simulink model "drone"  (Simulink 6.1)
settings: Solver=ode5  StartTime=0.0  StopTime=90  FixedStep=1e-3  RelTol=1e-3
values from neighbouring files (symbols this model uses):
  Aerodynamique =     [Test en vol.mat]
  Correcteur =     [Test en vol.mat]
  Mecanique =     [Test en vol.mat]
libraries: mblibv1 x43, simulink x26, aerolibtransform2 x4, electricdrivelib x1
(part 1 of 2)
settings Model: LastModifiedBy=Vincent
settings OptimizationCC: InlineParams=on
settings DebuggingCC: SolverPrmCheckMsg=warning
settings SimMechanicsCC: VisOnUpdateDiagram=on  VisDuringSimulation=on

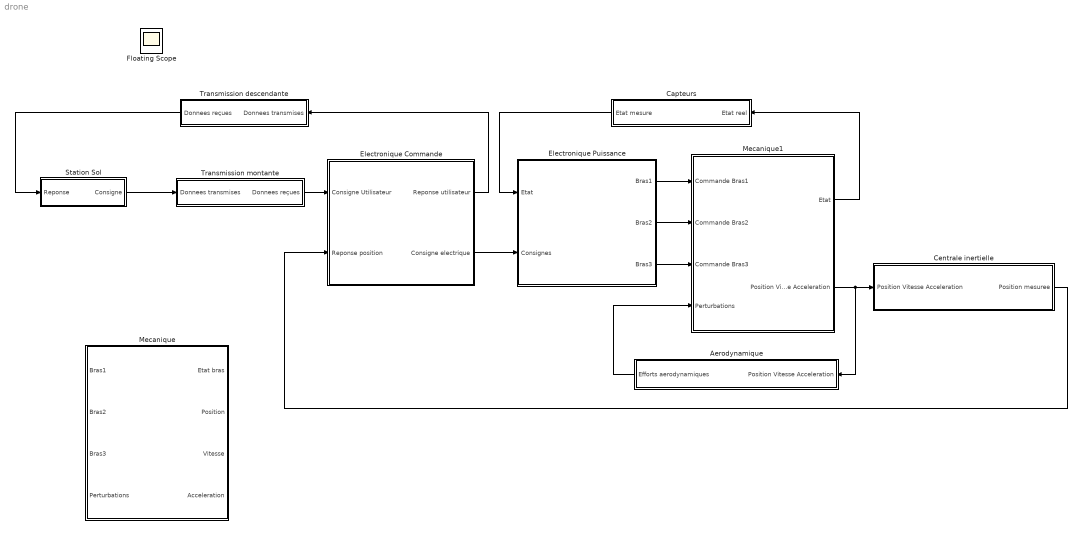
== system drone ==
  Aerodynamique : Subsystem  Orientation=left
  Capteurs : Subsystem  Orientation=left
  Centrale inertielle : Subsystem
  Electronique Commande : Subsystem
  Electronique Puissance : Subsystem
  Mecanique : Subsystem
  Mecanique1 : Subsystem
  Station Sol : Subsystem
  Transmission descendante : Subsystem  Orientation=left
  Transmission montante : Subsystem
  Floating Scope : Scope
      settings: Floating=on
  wires:
  Station Sol/1(Consigne) -> Transmission montante/1(Donnees transmises)
  Centrale inertielle/1(Position mesuree) -> Electronique Commande/2(Reponse position)
  Electronique Puissance/1(Bras1) -> Mecanique1/1(Commande Bras1)
  Electronique Puissance/3(Bras3) -> Mecanique1/3(Commande Bras3)
  Electronique Puissance/2(Bras2) -> Mecanique1/2(Commande Bras2)
  Electronique Commande/2(Consigne electrique) -> Electronique Puissance/2(Consignes)
  Aerodynamique/1(Efforts aerodynamiques) -> Mecanique1/4(Perturbations)
  Mecanique1/1(Etat) -> Capteurs/1(Etat reel)
  Capteurs/1(Etat mesure) -> Electronique Puissance/1(Etat)
  Transmission montante/1(Donnees reçues) -> Electronique Commande/1(Consigne Utilisateur)
  Electronique Commande/1(Reponse utilisateur) -> Transmission descendante/1(Donnees transmises)
  Transmission descendante/1(Donnees reçues) -> Station Sol/1(Reponse)
  Mecanique1/2(Position Vitesse Acceleration) -> Centrale inertielle/1(Position Vitesse Acceleration), Aerodynamique/1(Position Vitesse Acceleration)

== system drone/Aerodynamique ==
  Position Vitesse Acceleration : Inport  Port=1  LatchInput=off
  Bus Creator : BusCreator  DialogController=Simulink.DDGSource_Bus  Inputs=2
  Bus Selector : BusSelector  DialogController=Simulink.DDGSource_Bus  OutputSignals=x'y'z',pqr
  Coef frottement : Gain  Gain=-1*Aerodynamique.Resistance.F
  "Coef frottement " : Gain  Gain=-1*Aerodynamique.Resistance.C
  Efforts aerodynamiques : Outport
      settings: BusObject=perturbations
  wires:
  Position Vitesse Acceleration/1 -> Bus Selector/1
  Bus Selector/1 -> Coef frottement/1  "<x'y'z'>"
  Bus Selector/2 -> "Coef frottement "/1  "<pqr>"
  Coef frottement/1 -> Bus Creator/1  "forces aero"
  "Coef frottement "/1 -> Bus Creator/2  "couples aero"
  Bus Creator/1 -> Efforts aerodynamiques/1

== system drone/Capteurs ==
  Etat reel : Inport  Port=1  LatchInput=off
  Etat mesure : Outport
      settings: BusObject=perturbations
  wires:
  Etat reel/1 -> Etat mesure/1

== system drone/Centrale inertielle ==
  Position Vitesse Acceleration : Inport  Port=1  LatchInput=off
      settings: BusObject=couples_moteurs
  Bus Creator : BusCreator  DialogController=Simulink.DDGSource_Bus  Inputs=2
  Bus Selector : BusSelector  DialogController=Simulink.DDGSource_Bus  OutputSignals=xyz,dcm
  Direction Cosine Matrix  to Quaternions1 : aerolibtransform2/Direction Cosine Matrix  to Quaternions
  Position mesuree : Outport
      settings: BusObject=reponse_generale
  wires:
  Position Vitesse Acceleration/1 -> Bus Selector/1
  Bus Selector/2 -> Direction Cosine Matrix  to Quaternions1/1  "<dcm>"
  Bus Selector/1 -> Bus Creator/1  "<xyz>"
  Direction Cosine Matrix  to Quaternions1/1 -> Bus Creator/2  "quaternion"
  Bus Creator/1 -> Position mesuree/1

== system drone/Electronique Commande ==
  Consigne Utilisateur : Inport  Port=1  LatchInput=off
      settings: BusObject=consigne_generale
  Reponse position : Inport  Orientation=left  Port=2  LatchInput=off
      settings: BusObject=reponse_generale
  Adaptation Consigne : Subsystem
  Gestion Dynamique : Subsystem
  Reponse utilisateur : Outport  Orientation=left
      settings: BusObject=couples_moteurs
  Consigne electrique : Outport  Port=2
      settings: BusObject=couples_moteurs
  wires:
  Consigne Utilisateur/1 -> Gestion Dynamique/1(Consigne Etat)
  Adaptation Consigne/1(Fy1Fz1Fy2Fz2Fy3Fz3) -> Consigne electrique/1  "Consigne Efforts Adaptée"
  Gestion Dynamique/2(Consigne Efforts) -> Adaptation Consigne/1(FxFyFzCxCyCz)  "Consigne Efforts"
  Reponse position/1 -> Gestion Dynamique/2(Reponse Etat)
  Gestion Dynamique/1(Reponse Utilisateur) -> Reponse utilisateur/1

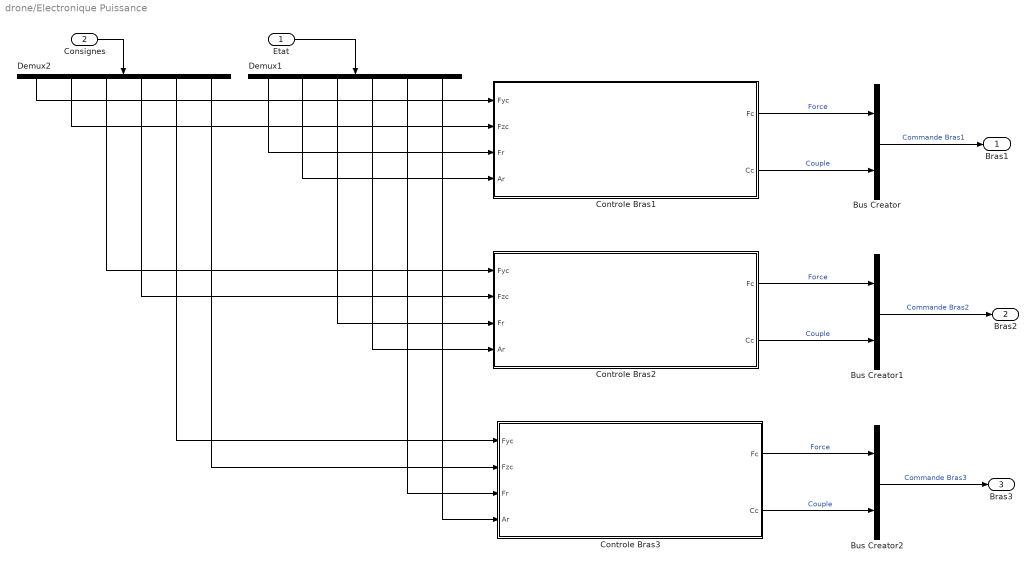
== system drone/Electronique Puissance ==
  Etat : Inport  Port=1  LatchInput=off
      settings: BusObject=consigne_generale
  Consignes : Inport  Port=2  LatchInput=off
      settings: BusObject=consigne_generale
  Bus Creator : BusCreator  DialogController=Simulink.DDGSource_Bus  Inputs=2
  Bus Creator1 : BusCreator  DialogController=Simulink.DDGSource_Bus  Inputs=2
  Bus Creator2 : BusCreator  DialogController=Simulink.DDGSource_Bus  Inputs=2
  Controle Bras1 : Subsystem
  Controle Bras2 : Subsystem
  Controle Bras3 : Subsystem
  Demux1 : Demux  Orientation=down  Outputs=6
  Demux2 : Demux  Orientation=down  Outputs=6
  Bras1 : Outport
      settings: BusObject=couples_moteurs
  Bras2 : Outport  Port=2
      settings: BusObject=couples_moteurs
  Bras3 : Outport  Port=3
      settings: BusObject=couples_moteurs
  wires:
  Bus Creator/1 -> Bras1/1  "Commande Bras1"
  Controle Bras1/1(Fc) -> Bus Creator/1  "Force"
  Controle Bras1/2(Cc) -> Bus Creator/2  "Couple"
  Controle Bras2/1(Fc) -> Bus Creator1/1  "Force"
  Bus Creator1/1 -> Bras2/1  "Commande Bras2"
  Controle Bras2/2(Cc) -> Bus Creator1/2  "Couple"
  Controle Bras3/1(Fc) -> Bus Creator2/1  "Force"
  Controle Bras3/2(Cc) -> Bus Creator2/2  "Couple"
  Bus Creator2/1 -> Bras3/1  "Commande Bras3"
  Etat/1 -> Demux1/1
  Demux1/1 -> Controle Bras1/3(Fr)
  Demux1/2 -> Controle Bras1/4(Ar)
  Consignes/1 -> Demux2/1
  Demux1/3 -> Controle Bras2/3(Fr)
  Demux1/4 -> Controle Bras2/4(Ar)
  Demux1/5 -> Controle Bras3/3(Fr)
  Demux1/6 -> Controle Bras3/4(Ar)
  Demux2/1 -> Controle Bras1/1(Fyc)
  Demux2/2 -> Controle Bras1/2(Fzc)
  Demux2/3 -> Controle Bras2/1(Fyc)
  Demux2/4 -> Controle Bras2/2(Fzc)
  Demux2/5 -> Controle Bras3/1(Fyc)
  Demux2/6 -> Controle Bras3/2(Fzc)

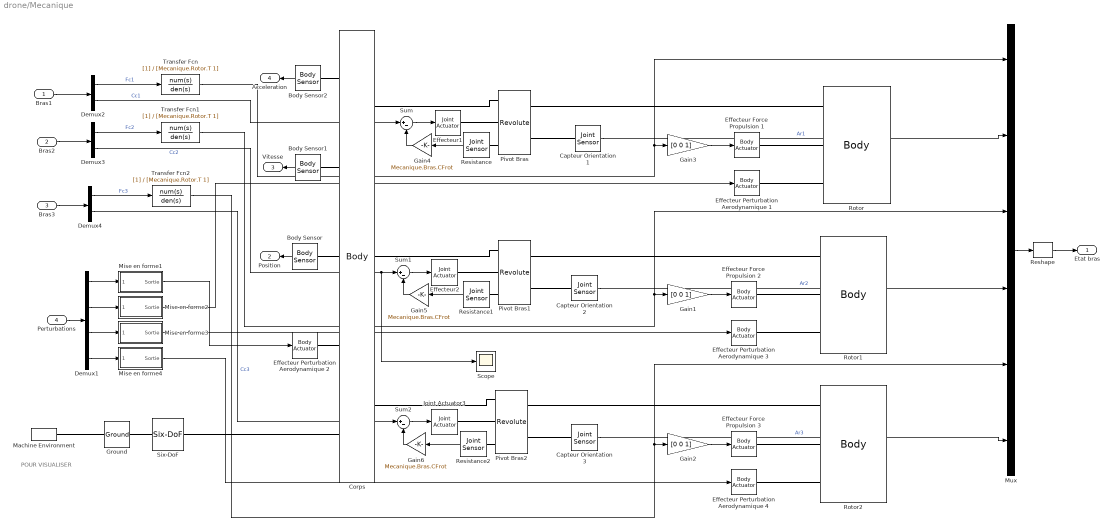
== system drone/Mecanique ==
  note: POUR VISUALISER
  Bras1 : Inport  Port=1  LatchInput=off
      settings: BusObject=couples_moteurs
  Bras2 : Inport  Port=2  LatchInput=off
      settings: BusObject=couples_moteurs
  Bras3 : Inport  Port=3  LatchInput=off
      settings: BusObject=couples_moteurs
  Perturbations : Inport  Port=4  LatchInput=off
      settings: BusObject=perturbations
  Body Sensor : mblibv1/Sensors &  Actuators/Body Sensor  Orientation=left  Opaque=on  PhysicalDomain=Mechanical  PortType=blob  Muxed=on  Pose=on  Angle=on  AngleUnits=deg  ArcVelocity=off  ArcVelocityUnits=deg/s  ArcAcceleration=off  ArcAccelerationUnits=deg/s^2  CoordPosition=on  CoordPositionUnits=m  Velocity=off  VelocityUnits=m/s  Acceleration=off  AccelerationUnits=m/s^2  Quaternion=on  QuaternionDT=off  QuaternionDDT=off  QuaternionUnits=off  OutputVector=[ 3 9 ]  ActiveIO=off  Width=12  DialogClass=MechanicalSensorBlock  ReferenceFrame=Absolute (World)
  Body Sensor1 : mblibv1/Sensors &  Actuators/Body Sensor  Orientation=left  Opaque=on  PhysicalDomain=Mechanical  PortType=blob  Muxed=on  Pose=off  Angle=on  AngleUnits=deg  ArcVelocity=on  ArcVelocityUnits=rad/s  ArcAcceleration=off  ArcAccelerationUnits=deg/s^2  CoordPosition=off  CoordPositionUnits=m  Velocity=on  VelocityUnits=m/s  Acceleration=off  AccelerationUnits=m/s^2  Quaternion=on  QuaternionDT=off  QuaternionDDT=off  QuaternionUnits=off  OutputVector=[ 3 3 ]  ActiveIO=off  Width=6  DialogClass=MechanicalSensorBlock  ReferenceFrame=Absolute (World)
  Body Sensor2 : mblibv1/Sensors &  Actuators/Body Sensor  Orientation=left  Opaque=on  PhysicalDomain=Mechanical  PortType=blob  Muxed=on  Pose=off  Angle=on  AngleUnits=deg  ArcVelocity=off  ArcVelocityUnits=deg/s  ArcAcceleration=on  ArcAccelerationUnits=rad/s^2  CoordPosition=off  CoordPositionUnits=m  Velocity=off  VelocityUnits=m/s  Acceleration=on  AccelerationUnits=m/s^2  Quaternion=on  QuaternionDT=off  QuaternionDDT=off  QuaternionUnits=off  OutputVector=[ 3 3 ]  ActiveIO=off  Width=6  DialogClass=MechanicalSensorBlock  ReferenceFrame=Absolute (World)
  Capteur Orientation 1 : mblibv1/Sensors &  Actuators/Joint Sensor  Opaque=on  PhysicalDomain=Mechanical  PortType=blob  Muxed=on  Pose=off  Angle=on  AngleUnits=rad  ArcVelocity=off  ArcVelocityUnits=rad/s  ArcAcceleration=off  ArcAccelerationUnits=rad/s^2  CoordPosition=on  CoordPositionUnits=m  Velocity=off  VelocityUnits=m/s  Acceleration=off  AccelerationUnits=m/s^2  Quaternion=on  QuaternionDT=off  QuaternionDDT=off  QuaternionUnits=off  OutputVector=[ 1 ]  ActiveIO=off  Width=1  DialogClass=MechanicalSensorBlock  Primitive=R1  Force=off  ForceUnits=N  Torque=off  TorqueUnits=N-m  ReferenceFrame=Absolute (INERTIAL)  ReactionSensedSide=Base  ReactionReferenceFrame=Local (Body CS)  ReactionForce=off  ReactionForceUnits=N  ReactionMoment=off  ReactionMomentUnits=N-m
  Capteur Orientation 2 : mblibv1/Sensors &  Actuators/Joint Sensor  Opaque=on  PhysicalDomain=Mechanical  PortType=blob  Muxed=on  Pose=off  Angle=on  AngleUnits=rad  ArcVelocity=off  ArcVelocityUnits=rad/s  ArcAcceleration=off  ArcAccelerationUnits=rad/s^2  CoordPosition=on  CoordPositionUnits=m  Velocity=off  VelocityUnits=m/s  Acceleration=off  AccelerationUnits=m/s^2  Quaternion=on  QuaternionDT=off  QuaternionDDT=off  QuaternionUnits=off  OutputVector=[ 1 ]  ActiveIO=off  Width=1  DialogClass=MechanicalSensorBlock  Primitive=R1  Force=off  ForceUnits=N  Torque=off  TorqueUnits=N-m  ReferenceFrame=Absolute (INERTIAL)  ReactionSensedSide=Base  ReactionReferenceFrame=Local (Body CS)  ReactionForce=off  ReactionForceUnits=N  ReactionMoment=off  ReactionMomentUnits=N-m
  Capteur Orientation 3 : mblibv1/Sensors &  Actuators/Joint Sensor  Opaque=on  PhysicalDomain=Mechanical  PortType=blob  Muxed=on  Pose=off  Angle=on  AngleUnits=rad  ArcVelocity=off  ArcVelocityUnits=rad/s  ArcAcceleration=off  ArcAccelerationUnits=rad/s^2  CoordPosition=on  CoordPositionUnits=m  Velocity=off  VelocityUnits=m/s  Acceleration=off  AccelerationUnits=m/s^2  Quaternion=on  QuaternionDT=off  QuaternionDDT=off  QuaternionUnits=off  OutputVector=[ 1 ]  ActiveIO=off  Width=1  DialogClass=MechanicalSensorBlock  Primitive=R1  Force=off  ForceUnits=N  Torque=off  TorqueUnits=N-m  ReferenceFrame=Absolute (INERTIAL)  ReactionSensedSide=Base  ReactionReferenceFrame=Local (Body CS)  ReactionForce=off  ReactionForceUnits=N  ReactionMoment=off  ReactionMomentUnits=N-m
  Corps : mblibv1/Bodies/Body  PhysicalDomain=mechanical  SubClassName=Unknown  LeftPortType=workingframe  RightPortType=workingframe  LConnTagsString=CS4|CS5|CS6|CS7|CG  RConnTagsString=CS1|CS2|CS3  DialogClass=MechanicalBodyBlock  Mass=Mecanique.Corps.Masse  MassUnits=kg  InertiaUnits=kg*m^2  Inertia=Mecanique.Corps.Inertie  Shape=Cylinder  ShapeDims=[1 1]  ShapeUnits=m  ShapeUse=false  Density=1  DensityUnits=kg/m^3  DensityUse=false  CG=Left$CG$[0 0 0]$ADJOINING$ADJOINING$m$[0 0 0]$Euler X-Y-Z$deg$ADJOINING$true  WorkingFrames=Right$CS1$[0 0 0]$CG$CG$m$[0 0 0]$Euler Z-Y-X$deg$CG$true#Right$CS2$[0 0 0]$CG$CG$m$[120 0 0]$Euler Z-Y-X$deg$CG$true#Right$CS3$[0 0 0]$CG$CG$m$[240 0 0]$Euler Z-Y-X$deg$CG$true#Left$CS4$[0 0 0]$CG$CG$m$[0 0 0]$Euler X-Y-Z$deg$WORLD$true#Left$CS5$[0 0 0]$CG$CG$m$[0 0 0]$Euler X-Y-Z$deg$WORLD$true#Left$CS6$[0 0 0]$CG$CG$m$[0 0 0]$Euler X-Y-Z$deg$WORLD$true#Left$CS7$[0 0 0]$CG$CG$m$[0 0 0]$Euler X-Y-Z$deg$WORLD$true
  Demux1 : Demux
  Demux2 : Demux  Outputs=2
  Demux3 : Demux  Outputs=2
  Demux4 : Demux  Outputs=2
  Effecteur Force Propulsion 1 : mblibv1/Sensors &  Actuators/Body Actuator  Opaque=on  PhysicalDomain=Mechanical  PortType=blob  ActuationStyle=Force  AngleUnits=deg  ArcVelocityUnits=deg/s  ArcAccelerationUnits=deg/s^2  CoordPositionUnits=m  VelocityUnits=m/s  AccelerationUnits=m/s^2  ForceUnits=N  TorqueUnits=N-m  ActiveIO=off  Width=3  DialogClass=MechanicalActuatorBlock  ReferenceFrame=Local (Body CS)  Angle=off  CoordPosition=on  Force=on  Torque=off
  Effecteur Force Propulsion 2 : mblibv1/Sensors &  Actuators/Body Actuator  Opaque=on  PhysicalDomain=Mechanical  PortType=blob  ActuationStyle=Force  AngleUnits=deg  ArcVelocityUnits=deg/s  ArcAccelerationUnits=deg/s^2  CoordPositionUnits=m  VelocityUnits=m/s  AccelerationUnits=m/s^2  ForceUnits=N  TorqueUnits=N-m  ActiveIO=off  Width=3  DialogClass=MechanicalActuatorBlock  ReferenceFrame=Local (Body CS)  Angle=off  CoordPosition=on  Force=on  Torque=off
  Effecteur Force Propulsion 3 : mblibv1/Sensors &  Actuators/Body Actuator  Opaque=on  PhysicalDomain=Mechanical  PortType=blob  ActuationStyle=Force  AngleUnits=deg  ArcVelocityUnits=deg/s  ArcAccelerationUnits=deg/s^2  CoordPositionUnits=m  VelocityUnits=m/s  AccelerationUnits=m/s^2  ForceUnits=N  TorqueUnits=N-m  ActiveIO=off  Width=3  DialogClass=MechanicalActuatorBlock  ReferenceFrame=Local (Body CS)  Angle=off  CoordPosition=on  Force=on  Torque=off
  Effecteur Perturbation Aerodynamique 1 : mblibv1/Sensors &  Actuators/Body Actuator  Opaque=on  PhysicalDomain=Mechanical  PortType=blob  ActuationStyle=Force  AngleUnits=deg  ArcVelocityUnits=deg/s  ArcAccelerationUnits=deg/s^2  CoordPositionUnits=m  VelocityUnits=m/s  AccelerationUnits=m/s^2  ForceUnits=N  TorqueUnits=N-m  ActiveIO=off  Width=6  DialogClass=MechanicalActuatorBlock  ReferenceFrame=Local (Body CS)  Angle=off  CoordPosition=on  Force=on  Torque=on
  Effecteur Perturbation Aerodynamique 2 : mblibv1/Sensors &  Actuators/Body Actuator  Opaque=on  PhysicalDomain=Mechanical  PortType=blob  ActuationStyle=Force  AngleUnits=deg  ArcVelocityUnits=deg/s  ArcAccelerationUnits=deg/s^2  CoordPositionUnits=m  VelocityUnits=m/s  AccelerationUnits=m/s^2  ForceUnits=N  TorqueUnits=N-m  ActiveIO=off  Width=6  DialogClass=MechanicalActuatorBlock  ReferenceFrame=Absolute (World)  Angle=off  CoordPosition=on  Force=on  Torque=on
  Effecteur Perturbation Aerodynamique 3 : mblibv1/Sensors &  Actuators/Body Actuator  Opaque=on  PhysicalDomain=Mechanical  PortType=blob  ActuationStyle=Force  AngleUnits=deg  ArcVelocityUnits=deg/s  ArcAccelerationUnits=deg/s^2  CoordPositionUnits=m  VelocityUnits=m/s  AccelerationUnits=m/s^2  ForceUnits=N  TorqueUnits=N-m  ActiveIO=off  Width=6  DialogClass=MechanicalActuatorBlock  ReferenceFrame=Local (Body CS)  Angle=off  CoordPosition=on  Force=on  Torque=on
  Effecteur Perturbation Aerodynamique 4 : mblibv1/Sensors &  Actuators/Body Actuator  Opaque=on  PhysicalDomain=Mechanical  PortType=blob  ActuationStyle=Force  AngleUnits=deg  ArcVelocityUnits=deg/s  ArcAccelerationUnits=deg/s^2  CoordPositionUnits=m  VelocityUnits=m/s  AccelerationUnits=m/s^2  ForceUnits=N  TorqueUnits=N-m  ActiveIO=off  Width=6  DialogClass=MechanicalActuatorBlock  ReferenceFrame=Local (Body CS)  Angle=off  CoordPosition=on  Force=on  Torque=on
  Effecteur1 : mblibv1/Sensors &  Actuators/Joint Actuator  Opaque=on  PhysicalDomain=Mechanical  PortType=blob  ActuationStyle=Force  AngleUnits=deg  ArcVelocityUnits=deg/s  ArcAccelerationUnits=deg/s^2  CoordPositionUnits=m  VelocityUnits=m/s  AccelerationUnits=m/s^2  ForceUnits=N  TorqueUnits=N-m  ActiveIO=off  Width=1  DialogClass=MechanicalActuatorBlock  Primitive=R1  ReferenceFrame=Absolute (INERTIAL)
  Effecteur2 : mblibv1/Sensors &  Actuators/Joint Actuator  Opaque=on  PhysicalDomain=Mechanical  PortType=blob  ActuationStyle=Force  AngleUnits=deg  ArcVelocityUnits=deg/s  ArcAccelerationUnits=deg/s^2  CoordPositionUnits=m  VelocityUnits=m/s  AccelerationUnits=m/s^2  ForceUnits=N  TorqueUnits=N-m  ActiveIO=off  Width=1  DialogClass=MechanicalActuatorBlock  Primitive=R1  ReferenceFrame=Absolute (INERTIAL)
  Gain1 : Gain  Gain=[0 0 1]
  Gain2 : Gain  Gain=[0 0 1]
  Gain3 : Gain  Gain=[0 0 1]
  Gain4 : Gain  Orientation=left  Gain=Mecanique.Bras.CFrot  SaturateOnIntegerOverflow=on
  Gain5 : Gain  Orientation=left  Gain=Mecanique.Bras.CFrot  SaturateOnIntegerOverflow=on
  Gain6 : Gain  Orientation=left  Gain=Mecanique.Bras.CFrot  SaturateOnIntegerOverflow=on
  Ground : mblibv1/Bodies/Ground  Opaque=on  LeftPortType=env  RightPortType=workingframe  PhysicalDomain=Mechanical  DialogClass=GroundBlock  CoordPosition=[0 0 0]  CoordPositionUnits=m  StateVectorMgrId=-1  MachineId=[0 0]  ShowEnvPort=on
  Joint Actuator3 : mblibv1/Sensors &  Actuators/Joint Actuator  Opaque=on  PhysicalDomain=Mechanical  PortType=blob  ActuationStyle=Force  AngleUnits=deg  ArcVelocityUnits=deg/s  ArcAccelerationUnits=deg/s^2  CoordPositionUnits=m  VelocityUnits=m/s  AccelerationUnits=m/s^2  ForceUnits=N  TorqueUnits=N-m  ActiveIO=off  Width=1  DialogClass=MechanicalActuatorBlock  Primitive=R1  ReferenceFrame=Absolute (INERTIAL)
  Machine Environment : mblibv1/Bodies/Machine Environment  Tag=Factory ground  DialogController=MECH.DialogSource  Opaque=on  PortType=env  PhysicalDomain=Mechanical  DialogTemplateClass=MECH.MachineEnvironment  SyncWhenCopied=off  Gravity=Environnement.Gravite  GravityUnits=m/s^2  GravityAsSignal=off  Dimensionality=3D Only  AnalysisType=Forward dynamics  LinearAssemblyTolerance=1e-3  LinearAssemblyToleranceUnits=m  AngularAssemblyTolerance=1e-3  AngularAssemblyToleranceUnits=rad  ConstraintSolverType=Stabilizing  ConstraintRelTolerance=1e-4  ConstraintAbsTolerance=1e-4  UseRobustSingularityHandling=off  StatePerturbationType=Fixed  PerturbationSize=1e-5  VisualizeMachine=on
  Mise en forme1 : Subsystem
  Mise en forme2 : Subsystem
  Mise en forme3 : Subsystem
  Mise en forme4 : Subsystem
  Mux : Mux  Inputs=6
  Pivot Bras : mblibv1/Joints/Revolute  PhysicalDomain=mechanical  SubClassName=Unknown  LeftPortType=blob  RightPortType=blob  LConnTagsString=__newl0|SA1|SA2  RConnTagsString=__newr0|SA1  NumSAPorts=3  CutJoint=off  MarkAsCut=off  Primitives=revolute  PrimitiveProps=R1$Base$[1 0 0]$revolute  DialogClass=JointBlock
  Pivot Bras1 : mblibv1/Joints/Revolute  PhysicalDomain=mechanical  SubClassName=Unknown  LeftPortType=blob  RightPortType=blob  LConnTagsString=__newl0|SA1|SA2  RConnTagsString=__newr0|SA1  NumSAPorts=3  CutJoint=off  MarkAsCut=off  Primitives=revolute  PrimitiveProps=R1$Base$[1 0 0]$revolute  DialogClass=JointBlock
  Pivot Bras2 : mblibv1/Joints/Revolute  PhysicalDomain=mechanical  SubClassName=Unknown  LeftPortType=blob  RightPortType=blob  LConnTagsString=__newl0|SA1|SA2  RConnTagsString=__newr0|SA1  NumSAPorts=3  CutJoint=off  MarkAsCut=off  Primitives=revolute  PrimitiveProps=R1$Base$[1 0 0]$revolute  DialogClass=JointBlock
  Reshape : simulink/Math Operations/Reshape  OutputDimensionality=1-D array  OutputDimensions=[1,1]
  Resistance : mblibv1/Sensors &  Actuators/Joint Sensor  Orientation=left  Opaque=on  PhysicalDomain=Mechanical  PortType=blob  Muxed=off  Pose=off  Angle=off  AngleUnits=rad  ArcVelocity=on  ArcVelocityUnits=rad/s  ArcAcceleration=off  ArcAccelerationUnits=rad/s^2  CoordPosition=on  CoordPositionUnits=m  Velocity=off  VelocityUnits=m/s  Acceleration=off  AccelerationUnits=m/s^2  Quaternion=on  QuaternionDT=off  QuaternionDDT=off  QuaternionUnits=off  OutputVector=[ 1 ]  ActiveIO=off  Width=1  DialogClass=MechanicalSensorBlock  Primitive=R1  Force=off  ForceUnits=N  Torque=off  TorqueUnits=N-m  ReferenceFrame=Absolute (INERTIAL)  ReactionSensedSide=Base  ReactionReferenceFrame=Local (Body CS)  ReactionForce=off  ReactionForceUnits=N  ReactionMoment=off  ReactionMomentUnits=N-m
  Resistance1 : mblibv1/Sensors &  Actuators/Joint Sensor  Orientation=left  Opaque=on  PhysicalDomain=Mechanical  PortType=blob  Muxed=off  Pose=off  Angle=off  AngleUnits=rad  ArcVelocity=on  ArcVelocityUnits=rad/s  ArcAcceleration=off  ArcAccelerationUnits=rad/s^2  CoordPosition=on  CoordPositionUnits=m  Velocity=off  VelocityUnits=m/s  Acceleration=off  AccelerationUnits=m/s^2  Quaternion=on  QuaternionDT=off  QuaternionDDT=off  QuaternionUnits=off  OutputVector=[ 1 ]  ActiveIO=off  Width=1  DialogClass=MechanicalSensorBlock  Primitive=R1  Force=off  ForceUnits=N  Torque=off  TorqueUnits=N-m  ReferenceFrame=Absolute (INERTIAL)  ReactionSensedSide=Base  ReactionReferenceFrame=Local (Body CS)  ReactionForce=off  ReactionForceUnits=N  ReactionMoment=off  ReactionMomentUnits=N-m
  Resistance2 : mblibv1/Sensors &  Actuators/Joint Sensor  Orientation=left  Opaque=on  PhysicalDomain=Mechanical  PortType=blob  Muxed=off  Pose=off  Angle=off  AngleUnits=rad  ArcVelocity=on  ArcVelocityUnits=rad/s  ArcAcceleration=off  ArcAccelerationUnits=rad/s^2  CoordPosition=on  CoordPositionUnits=m  Velocity=off  VelocityUnits=m/s  Acceleration=off  AccelerationUnits=m/s^2  Quaternion=on  QuaternionDT=off  QuaternionDDT=off  QuaternionUnits=off  OutputVector=[ 1 ]  ActiveIO=off  Width=1  DialogClass=MechanicalSensorBlock  Primitive=R1  Force=off  ForceUnits=N  Torque=off  TorqueUnits=N-m  ReferenceFrame=Absolute (INERTIAL)  ReactionSensedSide=Base  ReactionReferenceFrame=Local (Body CS)  ReactionForce=off  ReactionForceUnits=N  ReactionMoment=off  ReactionMomentUnits=N-m
  Rotor : mblibv1/Bodies/Body  PhysicalDomain=mechanical  SubClassName=Unknown  LeftPortType=workingframe  RightPortType=workingframe  LConnTagsString=CS1|CS2|CS3  DialogClass=MechanicalBodyBlock  Mass=Mecanique.Bras.Masse  MassUnits=kg  InertiaUnits=kg*m^2  Inertia=Mecanique.Bras.Inertie  Shape=Cylinder  ShapeDims=[1 1]  ShapeUnits=m  ShapeUse=false  Density=1  DensityUnits=kg/m^3  DensityUse=false  CG=Left$CG$Mecanique.Longeur*[1 0 0]$CS1$CS1$m$[0 0 0]$Euler X-Y-Z$deg$CS1$false  WorkingFrames=Left$CS1$[0 0 0]$ADJOINING$ADJOINING$m$[0 0 0]$Euler X-Y-Z$deg$ADJOINING$true#Left$CS2$Mecanique.Longeur*[1 0 0]$CS1$CS1$m$[0 0 0]$Euler X-Y-Z$deg$CS1$true#Left$CS3$Mecanique.Longeur*[1 0 0]$CS1$CS1$m$[0 0 0]$Euler X-Y-Z$deg$CS1$true
  Rotor1 : mblibv1/Bodies/Body  PhysicalDomain=mechanical  SubClassName=Unknown  LeftPortType=workingframe  RightPortType=workingframe  LConnTagsString=CS1|CS2|CS3  DialogClass=MechanicalBodyBlock  Mass=Mecanique.Bras.Masse  MassUnits=kg  InertiaUnits=kg*m^2  Inertia=Mecanique.Bras.Inertie  Shape=Cylinder  ShapeDims=[1 1]  ShapeUnits=m  ShapeUse=false  Density=1  DensityUnits=kg/m^3  DensityUse=false  CG=Left$CG$Mecanique.Longeur*[1 0 0]$CS1$CS1$m$[0 0 0]$Euler X-Y-Z$deg$CS1$false  WorkingFrames=Left$CS1$[0 0 0]$ADJOINING$ADJOINING$m$[0 0 0]$Euler X-Y-Z$deg$ADJOINING$true#Left$CS2$Mecanique.Longeur*[1 0 0]$CS1$CS1$m$[0 0 0]$Euler X-Y-Z$deg$CS1$true#Left$CS3$Mecanique.Longeur*[1 0 0]$CS1$CS1$m$[0 0 0]$Euler X-Y-Z$deg$CS1$true
  Rotor2 : mblibv1/Bodies/Body  PhysicalDomain=mechanical  SubClassName=Unknown  LeftPortType=workingframe  RightPortType=workingframe  LConnTagsString=CS1|CS2|CS3  DialogClass=MechanicalBodyBlock  Mass=Mecanique.Bras.Masse  MassUnits=kg  InertiaUnits=kg*m^2  Inertia=Mecanique.Bras.Inertie  Shape=Cylinder  ShapeDims=[1 1]  ShapeUnits=m  ShapeUse=false  Density=1  DensityUnits=kg/m^3  DensityUse=false  CG=Left$CG$Mecanique.Longeur*[1 0 0]$CS1$CS1$m$[0 0 0]$Euler X-Y-Z$deg$CS1$false  WorkingFrames=Left$CS1$[0 0 0]$ADJOINING$ADJOINING$m$[0 0 0]$Euler X-Y-Z$deg$ADJOINING$true#Left$CS2$Mecanique.Longeur*[1 0 0]$CS1$CS1$m$[0 0 0]$Euler X-Y-Z$deg$CS1$true#Left$CS3$Mecanique.Longeur*[1 0 0]$CS1$CS1$m$[0 0 0]$Euler X-Y-Z$deg$CS1$true
  Scope : Scope
      settings: YMin=-0.5  YMax=0.5  SaveName=ScopeData8
  Six-DoF : mblibv1/Joints/Six-DoF  PhysicalDomain=mechanical  SubClassName=Unknown  LeftPortType=blob  RightPortType=blob  LConnTagsString=__newl0  RConnTagsString=__newr0  NumSAPorts=0  CutJoint=off  MarkAsCut=off  Primitives=prismatic_prismatic_prismatic_spherical  PrimitiveProps=P1$INERTIAL$[1 0 0]$prismatic#P2$INERTIAL$[0 1 0]$prismatic#P3$INERTIAL$[0 0 1]$prismatic#S$INERTIAL$[0 0 0]$spherical  DialogClass=JointBlock
  Sum : Sum  Inputs=|+-
  Sum1 : Sum  Inputs=|+-
  Sum2 : Sum  Inputs=|+-
  Transfer Fcn : TransferFcn  Denominator=[Mecanique.Rotor.T 1]
  Transfer Fcn1 : TransferFcn  Denominator=[Mecanique.Rotor.T 1]
  Transfer Fcn2 : TransferFcn  Denominator=[Mecanique.Rotor.T 1]
  Etat bras : Outport
      settings: BusObject=angles_moteurs
  Position : Outport  Orientation=left  Port=2
      settings: BusObject=angles_moteurs
  Vitesse : Outport  Orientation=left  Port=3
      settings: BusObject=angles_moteurs
  Acceleration : Outport  Orientation=left  Port=4
      settings: BusObject=angles_moteurs
  wires:
  Bras1/1 -> Demux2/1
  Demux2/2 -> Sum/1  "Cc1"
  Demux2/1 -> Transfer Fcn/1  "Fc1"
  Demux3/2 -> Sum1/1, Scope/1  "Cc2"
  Demux3/1 -> Transfer Fcn1/1  "Fc2"
  Demux4/1 -> Transfer Fcn2/1  "Fc3"
  Demux4/2 -> Sum2/1  "Cc3"
  Reshape/1 -> Etat bras/1
  Capteur Orientation 3/1 -> Mux/6  "Ar3"
  Capteur Orientation 2/1 -> Mux/4  "Ar2"
  Capteur Orientation 1/1 -> Mux/2  "Ar1"
  Mux/1 -> Reshape/1
  Gain2/1 -> Effecteur Force Propulsion 3/1
  Gain1/1 -> Effecteur Force Propulsion 2/1
  Gain3/1 -> Effecteur Force Propulsion 1/1
  Perturbations/1 -> Demux1/1
  Demux1/2 -> Mise en forme2/1(Entree)
  Demux1/3 -> Mise en forme3/1(Entree)
  Demux1/4 -> Mise en forme4/1(Entree)
  Demux1/1 -> Mise en forme1/1(Entree)
  Sum/1 -> Effecteur1/1
  Resistance/1 -> Gain4/1
  Gain4/1 -> Sum/2
  Gain5/1 -> Sum1/2
  Resistance1/1 -> Gain5/1
  Sum1/1 -> Effecteur2/1
  Gain6/1 -> Sum2/2
  Resistance2/1 -> Gain6/1
  Sum2/1 -> Joint Actuator3/1
  Transfer Fcn/1 -> Mux/1, Gain3/1
  Transfer Fcn1/1 -> Mux/3, Gain1/1
  Transfer Fcn2/1 -> Mux/5, Gain2/1
  Body Sensor/1 -> Position/1
  Body Sensor1/1 -> Vitesse/1
  Body Sensor2/1 -> Acceleration/1
  Mise en forme1/1(Sortie) -> Effecteur Perturbation Aerodynamique 2/1
  Mise en forme2/1(Sortie) -> Effecteur Perturbation Aerodynamique 1/1
  Mise en forme3/1(Sortie) -> Effecteur Perturbation Aerodynamique 3/1
  Mise en forme4/1(Sortie) -> Effecteur Perturbation Aerodynamique 4/1
  Bras3/1 -> Demux4/1
  Bras2/1 -> Demux3/1
  connections:
  Corps/RConn1 -- Pivot Bras/LConn1
  Pivot Bras/RConn1 -- Rotor/LConn1
  Effecteur Force Propulsion 1/RConn1 -- Rotor/LConn2
  Effecteur Perturbation Aerodynamique 1/RConn1 -- Rotor/LConn3
  Pivot Bras/RConn2 -- Capteur Orientation 1/LConn1
  Ground/RConn1 -- Six-DoF/LConn1
  Six-DoF/RConn1 -- Corps/LConn5
  Machine Environment/RConn1 -- Ground/LConn1
  Effecteur1/RConn1 -- Pivot Bras/LConn2
  Pivot Bras1/RConn1 -- Rotor1/LConn1
  Effecteur Force Propulsion 2/RConn1 -- Rotor1/LConn2
  Effecteur Perturbation Aerodynamique 3/RConn1 -- Rotor1/LConn3
  Pivot Bras1/RConn2 -- Capteur Orientation 2/LConn1
  Effecteur2/RConn1 -- Pivot Bras1/LConn2
  Pivot Bras2/RConn1 -- Rotor2/LConn1
  Effecteur Force Propulsion 3/RConn1 -- Rotor2/LConn2
  Effecteur Perturbation Aerodynamique 4/RConn1 -- Rotor2/LConn3
  Pivot Bras2/RConn2 -- Capteur Orientation 3/LConn1
  Joint Actuator3/RConn1 -- Pivot Bras2/LConn2
  Corps/RConn2 -- Pivot Bras1/LConn1
  Corps/RConn3 -- Pivot Bras2/LConn1
  Pivot Bras/LConn3 -- Resistance/LConn1
  Pivot Bras1/LConn3 -- Resistance1/LConn1
  Pivot Bras2/LConn3 -- Resistance2/LConn1
  Effecteur Perturbation Aerodynamique 2/RConn1 -- Corps/LConn4
  Corps/LConn3 -- Body Sensor/LConn1
  Body Sensor1/LConn1 -- Corps/LConn2
  Body Sensor2/LConn1 -- Corps/LConn1

== system drone/Mecanique1 ==
  Commande Bras1 : Inport  Port=1  LatchInput=off
      settings: BusObject=couples_moteurs
  Commande Bras2 : Inport  Port=2  LatchInput=off
      settings: BusObject=couples_moteurs
  Commande Bras3 : Inport  Port=3  LatchInput=off
      settings: BusObject=couples_moteurs
  Perturbations : Inport  Port=4  LatchInput=off
      settings: BusObject=perturbations
  Air : Subsystem  Orientation=left
  Bras1 : Subsystem
  Bus Selector : BusSelector  DialogController=Simulink.DDGSource_Bus  OutputSignals=forces aero,couples aero
  Corps : Subsystem  Orientation=left
  Environnement : Subsystem  Orientation=left
  Etat : Outport
  Position Vitesse Acceleration : Outport  Orientation=left  Port=2
  wires:
  Corps/1(Position Vitesse Acceleration) -> Position Vitesse Acceleration/1
  Commande Bras1/1 -> Bras1/1(Commande)
  Perturbations/1 -> Bus Selector/1
  connections:
  Bras1/LConn1 -- Corps/LConn1
  Environnement/LConn1 -- Corps/RConn2
  Air/LConn1 -- Corps/RConn1

== system drone/Station Sol ==
  Reponse : Inport  Orientation=left  Port=1  LatchInput=off
  Demux : Demux
  Demux1 : Demux  Outputs=6
  Euler Angles to Quaternions : aerolibtransform2/Euler Angles to Quaternions
  Mux : Mux  Inputs=7
  Mux1 : Mux  Inputs=3
  Reshape2 : simulink/Math Operations/Reshape  OutputDimensionality=1-D array  OutputDimensions=[1,1]
  Scope : Scope
      settings: SaveName=ScopeData10
  Trajet predefini : FromFile  FileName=trajet.mat  SampleTime=0
  Consigne : Outport
      settings: BusObject=consigne_generale
  wires:
  Mux/1 -> Reshape2/1
  Reshape2/1 -> Consigne/1
  Demux1/1 -> Mux/1
  Demux1/2 -> Mux/2
  Demux1/3 -> Mux/3
  Demux1/4 -> Mux1/1
  Demux1/5 -> Mux1/2
  Demux1/6 -> Mux1/3
  Mux1/1 -> Euler Angles to Quaternions/1
  Demux/4 -> Mux/7
  Euler Angles to Quaternions/1 -> Demux/1
  Demux/3 -> Mux/6
  Demux/2 -> Mux/5
  Demux/1 -> Mux/4
  Trajet predefini/1 -> Demux1/1
  Reponse/1 -> Scope/1

== system drone/Transmission descendante ==
  Donnees transmises : Inport  Port=1  LatchInput=off
  Delai de transmission : VariableTransportDelay  MaximumDelay=10
  Valeur du delai : Constant  Value=0.01
  Donnees reçues : Outport
      settings: BusObject=perturbations
  wires:
  Donnees transmises/1 -> Delai de transmission/1
  Delai de transmission/1 -> Donnees reçues/1
  Valeur du delai/1 -> Delai de transmission/2

== system drone/Transmission montante ==
  Donnees transmises : Inport  Port=1  LatchInput=off
  Delai de transmission : VariableTransportDelay  MaximumDelay=10
  Valeur du delai : Constant  Value=0.01
  Donnees reçues : Outport
      settings: BusObject=perturbations
  wires:
  Donnees transmises/1 -> Delai de transmission/1
  Delai de transmission/1 -> Donnees reçues/1
  Valeur du delai/1 -> Delai de transmission/2

== system drone/Electronique Commande/Adaptation Consigne ==
  FxFyFzCxCyCz : Inport  Port=1  LatchInput=off
  Matrice Correction : Constant  Value=[-1 -1 1 1/Mecanique.Longeur 1/Mecanique.Longeur 1/Mecanique.Longeur]
  Matrice Transformation : Constant  Value=(1/3)*[0 2 0 0 0 1; 0 0 1 0 2 0; -sqrt(3) -1 0 0 0 1; 0 0 1 -sqrt(3) -1 0; sqrt(3) -1 0 0 0 1; 0 0 1 sqrt(3) -1 0]  VectorParams1D=off
  Product : Product  Multiplication=Matrix(*)  RndMeth=Zero
  Product1 : Product  RndMeth=Zero
  Fy1Fz1Fy2Fz2Fy3Fz3 : Outport
  wires:
  Product/1 -> Fy1Fz1Fy2Fz2Fy3Fz3/1
  Matrice Transformation/1 -> Product/1
  Matrice Correction/1 -> Product1/2
  FxFyFzCxCyCz/1 -> Product1/1
  Product1/1 -> Product/2

== system drone/Electronique Commande/Gestion Dynamique ==
  Consigne Etat : Inport  Port=1  LatchInput=off
  Reponse Etat : Inport  Port=2  LatchInput=off
  Calcul Attitude : Subsystem
  Calcul Position : Subsystem
  Concatenation composantes : Subsystem
  Extraction attitude : Subsystem
  Separation composantes et erreur de position : Subsystem
  Reponse Utilisateur : Outport
  Consigne Efforts : Outport  Port=2
  wires:
  Consigne Etat/1 -> Separation composantes et erreur de position/1(Consigne)
  Concatenation composantes/1(Ordres) -> Consigne Efforts/1
  Calcul Position/1(Ordres Position) -> Concatenation composantes/1(Ordres position)
  Calcul Attitude/1(Ordres Attitude) -> Concatenation composantes/2(Ordres attitude)
  Separation composantes et erreur de position/1(Erreur Position) -> Calcul Position/1(Erreur Position)
  Separation composantes et erreur de position/2(Erreur Attitude) -> Calcul Attitude/1(Erreur Attitude)
  Reponse Etat/1 -> Separation composantes et erreur de position/2(Reponse), Extraction attitude/1(Etat)
  Extraction attitude/1(Attitude) -> Calcul Position/2(Attitude), Calcul Attitude/2(Attitude)

== system drone/Electronique Puissance/Controle Bras1 ==
  Fyc : Inport  Port=1  LatchInput=off
  Fzc : Inport  Port=2  LatchInput=off
  Fr : Inport  Port=3  LatchInput=off
  Ar : Inport  Port=4  LatchInput=off
  Carte electronique : Subsystem
  Moteur orientation : Subsystem
  Moteur propulsion : Subsystem
  Fc : Outport
  Cc : Outport  Port=2
  wires:
  Fyc/1 -> Carte electronique/1(Fyc)
  Fzc/1 -> Carte electronique/2(Fzc)
  Ar/1 -> Carte electronique/4(Ar)
  Fr/1 -> Carte electronique/3(Fr)
  Carte electronique/1(Fc) -> Moteur propulsion/1(Fz)
  Moteur propulsion/1(Couple) -> Fc/1
  Carte electronique/2(Cc) -> Moteur orientation/1(Fz)
  Moteur orientation/1(Couple) -> Cc/1

== system drone/Electronique Puissance/Controle Bras2 ==
  Fyc : Inport  Port=1  LatchInput=off
  Fzc : Inport  Port=2  LatchInput=off
  Fr : Inport  Port=3  LatchInput=off
  Ar : Inport  Port=4  LatchInput=off
  Carte electronique : Subsystem
  Moteur orientation : Subsystem
  Moteur propulsion : Subsystem
  Fc : Outport
  Cc : Outport  Port=2
  wires:
  Fyc/1 -> Carte electronique/1(Fyc)
  Fzc/1 -> Carte electronique/2(Fzc)
  Ar/1 -> Carte electronique/4(Ar)
  Fr/1 -> Carte electronique/3(Fr)
  Carte electronique/1(Fc) -> Moteur propulsion/1(Fz)
  Moteur propulsion/1(Couple) -> Fc/1
  Carte electronique/2(Cc) -> Moteur orientation/1(Fz)
  Moteur orientation/1(Couple) -> Cc/1

== system drone/Electronique Puissance/Controle Bras3 ==
  Fyc : Inport  Port=1  LatchInput=off
  Fzc : Inport  Port=2  LatchInput=off
  Fr : Inport  Port=3  LatchInput=off
  Ar : Inport  Port=4  LatchInput=off
  Carte electronique : Subsystem
  Moteur orientation : Subsystem
  Moteur propulsion : Subsystem
  Fc : Outport
  Cc : Outport  Port=2
  wires:
  Fyc/1 -> Carte electronique/1(Fyc)
  Fzc/1 -> Carte electronique/2(Fzc)
  Ar/1 -> Carte electronique/4(Ar)
  Fr/1 -> Carte electronique/3(Fr)
  Carte electronique/1(Fc) -> Moteur propulsion/1(Fz)
  Moteur propulsion/1(Couple) -> Fc/1
  Carte electronique/2(Cc) -> Moteur orientation/1(Fz)
  Moteur orientation/1(Couple) -> Cc/1

== system drone/Mecanique/Mise en forme1 ==
  Entree : Inport  Port=1  LatchInput=off
  Demux2 : Demux  Outputs=2
  Mux1 : Mux  Inputs=2
  Reshape1 : simulink/Math Operations/Reshape  OutputDimensionality=1-D array  OutputDimensions=[1,1]
  Sortie : Outport
  wires:
  Entree/1 -> Demux2/1
  Mux1/1 -> Reshape1/1
  Demux2/2 -> Mux1/1
  Demux2/1 -> Mux1/2
  Reshape1/1 -> Sortie/1

== system drone/Mecanique/Mise en forme2 ==
  Entree : Inport  Port=1  LatchInput=off
  Demux2 : Demux  Outputs=2
  Mux1 : Mux  Inputs=2
  Reshape1 : simulink/Math Operations/Reshape  OutputDimensionality=1-D array  OutputDimensions=[1,1]
  Sortie : Outport
  wires:
  Reshape1/1 -> Sortie/1
  Demux2/1 -> Mux1/2
  Demux2/2 -> Mux1/1
  Mux1/1 -> Reshape1/1
  Entree/1 -> Demux2/1

== system drone/Mecanique/Mise en forme3 ==
  Entree : Inport  Port=1  LatchInput=off
  Demux2 : Demux  Outputs=2
  Mux1 : Mux  Inputs=2
  Reshape1 : simulink/Math Operations/Reshape  OutputDimensionality=1-D array  OutputDimensions=[1,1]
  Sortie : Outport
  wires:
  Entree/1 -> Demux2/1
  Mux1/1 -> Reshape1/1
  Demux2/2 -> Mux1/1
  Demux2/1 -> Mux1/2
  Reshape1/1 -> Sortie/1

== system drone/Mecanique/Mise en forme4 ==
  Entree : Inport  Port=1  LatchInput=off
  Demux2 : Demux  Outputs=2
  Mux1 : Mux  Inputs=2
  Reshape1 : simulink/Math Operations/Reshape  OutputDimensionality=1-D array  OutputDimensions=[1,1]
  Sortie : Outport
  wires:
  Reshape1/1 -> Sortie/1
  Demux2/1 -> Mux1/2
  Demux2/2 -> Mux1/1
  Mux1/1 -> Reshape1/1
  Entree/1 -> Demux2/1

== system drone/Mecanique1/Air ==
  Efforts : Inport  Port=1  LatchInput=off
  Corps : PMIOPort  Tag=PMCPort  Orientation=left  Port=1  Side=Left

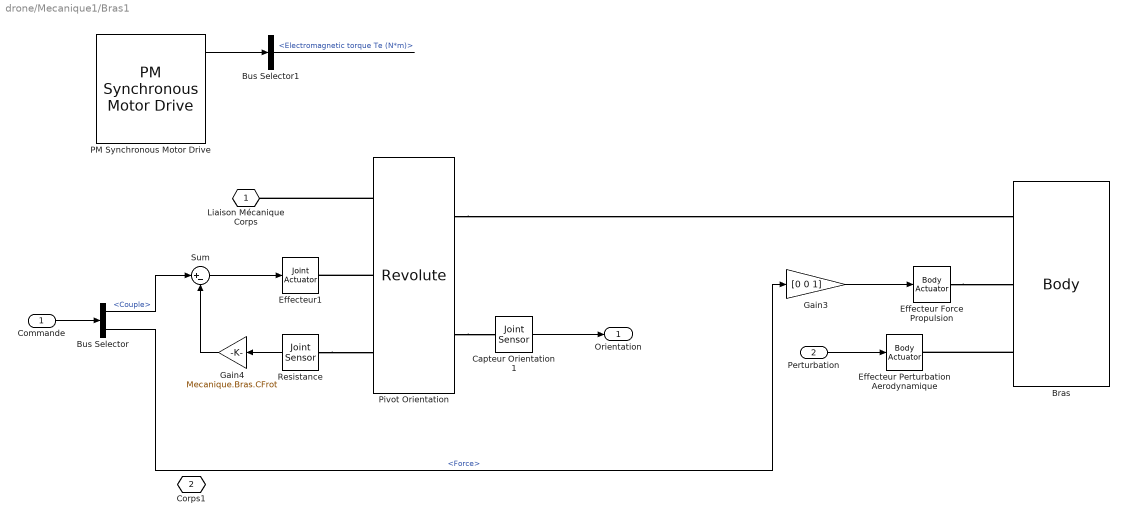
== system drone/Mecanique1/Bras1 ==
  Commande : Inport  Port=1  LatchInput=off
  Perturbation : Inport  Port=2  LatchInput=off
  Bras : mblibv1/Bodies/Body  PhysicalDomain=mechanical  SubClassName=Unknown  LeftPortType=workingframe  RightPortType=workingframe  LConnTagsString=CS1|CS2|CS3  DialogClass=MechanicalBodyBlock  Mass=Mecanique.Bras.Masse  MassUnits=kg  InertiaUnits=kg*m^2  Inertia=Mecanique.Bras.Inertie  Shape=Cylinder  ShapeDims=[1 1]  ShapeUnits=m  ShapeUse=false  Density=1  DensityUnits=kg/m^3  DensityUse=false  CG=Left$CG$Mecanique.Longeur*[1 0 0]$CS1$CS1$m$[0 0 0]$Euler X-Y-Z$deg$CS1$false  WorkingFrames=Left$CS1$[0 0 0]$ADJOINING$ADJOINING$m$[0 0 0]$Euler X-Y-Z$deg$ADJOINING$true#Left$CS2$Mecanique.Longeur*[1 0 0]$CS1$CS1$m$[0 0 0]$Euler X-Y-Z$deg$CS1$true#Left$CS3$Mecanique.Longeur*[1 0 0]$CS1$CS1$m$[0 0 0]$Euler X-Y-Z$deg$CS1$true
  Bus Selector : BusSelector  DialogController=Simulink.DDGSource_Bus  OutputSignals=Couple,Force
  Bus Selector1 : BusSelector  DialogController=Simulink.DDGSource_Bus  OutputSignals=Electromagnetic torque Te (N*m)
  Capteur Orientation 1 : mblibv1/Sensors &  Actuators/Joint Sensor  Opaque=on  PhysicalDomain=Mechanical  PortType=blob  Muxed=on  Pose=off  Angle=on  AngleUnits=rad  ArcVelocity=off  ArcVelocityUnits=rad/s  ArcAcceleration=off  ArcAccelerationUnits=rad/s^2  CoordPosition=on  CoordPositionUnits=m  Velocity=off  VelocityUnits=m/s  Acceleration=off  AccelerationUnits=m/s^2  Quaternion=on  QuaternionDT=off  QuaternionDDT=off  QuaternionUnits=off  OutputVector=[ 1 ]  ActiveIO=off  Width=1  DialogClass=MechanicalSensorBlock  Primitive=R1  Force=off  ForceUnits=N  Torque=off  TorqueUnits=N-m  ReferenceFrame=Absolute (INERTIAL)  ReactionSensedSide=Base  ReactionReferenceFrame=Local (Body CS)  ReactionForce=off  ReactionForceUnits=N  ReactionMoment=off  ReactionMomentUnits=N-m
  Effecteur Force Propulsion : mblibv1/Sensors &  Actuators/Body Actuator  Opaque=on  PhysicalDomain=Mechanical  PortType=blob  ActuationStyle=Force  AngleUnits=deg  ArcVelocityUnits=deg/s  ArcAccelerationUnits=deg/s^2  CoordPositionUnits=m  VelocityUnits=m/s  AccelerationUnits=m/s^2  ForceUnits=N  TorqueUnits=N-m  ActiveIO=off  Width=3  DialogClass=MechanicalActuatorBlock  ReferenceFrame=Local (Body CS)  Angle=off  CoordPosition=on  Force=on  Torque=off
  "Effecteur Perturbation Aerodynamique " : mblibv1/Sensors &  Actuators/Body Actuator  Opaque=on  PhysicalDomain=Mechanical  PortType=blob  ActuationStyle=Force  AngleUnits=deg  ArcVelocityUnits=deg/s  ArcAccelerationUnits=deg/s^2  CoordPositionUnits=m  VelocityUnits=m/s  AccelerationUnits=m/s^2  ForceUnits=N  TorqueUnits=N-m  ActiveIO=off  Width=6  DialogClass=MechanicalActuatorBlock  ReferenceFrame=Local (Body CS)  Angle=off  CoordPosition=on  Force=on  Torque=on
  Effecteur1 : mblibv1/Sensors &  Actuators/Joint Actuator  Opaque=on  PhysicalDomain=Mechanical  PortType=blob  ActuationStyle=Force  AngleUnits=deg  ArcVelocityUnits=deg/s  ArcAccelerationUnits=deg/s^2  CoordPositionUnits=m  VelocityUnits=m/s  AccelerationUnits=m/s^2  ForceUnits=N  TorqueUnits=N-m  ActiveIO=off  Width=1  DialogClass=MechanicalActuatorBlock  Primitive=R1  ReferenceFrame=Absolute (INERTIAL)
  Gain3 : Gain  Gain=[0 0 1]
  Gain4 : Gain  Orientation=left  Gain=Mecanique.Bras.CFrot  SaturateOnIntegerOverflow=on
  PM Synchronous Motor Drive : electricdrivelib/AC drives/PM Synchronous Motor Drive
  Pivot Orientation : mblibv1/Joints/Revolute  PhysicalDomain=mechanical  SubClassName=Unknown  LeftPortType=blob  RightPortType=blob  LConnTagsString=__newl0|SA1|SA2  RConnTagsString=__newr0|SA1  NumSAPorts=3  CutJoint=off  MarkAsCut=off  Primitives=revolute  PrimitiveProps=R1$Base$[1 0 0]$revolute  DialogClass=JointBlock
  Resistance : mblibv1/Sensors &  Actuators/Joint Sensor  Orientation=left  Opaque=on  PhysicalDomain=Mechanical  PortType=blob  Muxed=off  Pose=off  Angle=off  AngleUnits=rad  ArcVelocity=on  ArcVelocityUnits=rad/s  ArcAcceleration=off  ArcAccelerationUnits=rad/s^2  CoordPosition=on  CoordPositionUnits=m  Velocity=off  VelocityUnits=m/s  Acceleration=off  AccelerationUnits=m/s^2  Quaternion=on  QuaternionDT=off  QuaternionDDT=off  QuaternionUnits=off  OutputVector=[ 1 ]  ActiveIO=off  Width=1  DialogClass=MechanicalSensorBlock  Primitive=R1  Force=off  ForceUnits=N  Torque=off  TorqueUnits=N-m  ReferenceFrame=Absolute (INERTIAL)  ReactionSensedSide=Base  ReactionReferenceFrame=Local (Body CS)  ReactionForce=off  ReactionForceUnits=N  ReactionMoment=off  ReactionMomentUnits=N-m
  Sum : Sum  Inputs=|+-
  Liaison Mécanique Corps : PMIOPort  Tag=PMCPort  Port=1  Side=Left
  Corps1 : PMIOPort  Tag=PMCPort  Port=2  Side=Right
  Orientation : Outport
  wires:
  Resistance/1 -> Gain4/1
  Gain4/1 -> Sum/2
  Sum/1 -> Effecteur1/1
  Perturbation/1 -> "Effecteur Perturbation Aerodynamique "/1
  Capteur Orientation 1/1 -> Orientation/1
  Gain3/1 -> Effecteur Force Propulsion/1
  Commande/1 -> Bus Selector/1
  Bus Selector/1 -> Sum/1  "<Couple>"
  Bus Selector/2 -> Gain3/1  "<Force>"
  PM Synchronous Motor Drive/1 -> Bus Selector1/1
  Bus Selector1/1 -> ?  "<Electromagnetic torque Te (N*m)>"
  connections:
  Resistance/LConn1 -- Pivot Orientation/LConn3
  Pivot Orientation/LConn2 -- Effecteur1/RConn1
  Pivot Orientation/LConn1 -- Liaison Mécanique Corps/RConn1
  Pivot Orientation/RConn1 -- Bras/LConn1
  Bras/LConn3 -- "Effecteur Perturbation Aerodynamique "/RConn1
  Pivot Orientation/RConn2 -- Capteur Orientation 1/LConn1
  Effecteur Force Propulsion/RConn1 -- Bras/LConn2

== system drone/Mecanique1/Corps ==
  Body Sensor : mblibv1/Sensors &  Actuators/Body Sensor  Orientation=left  Opaque=on  PhysicalDomain=Mechanical  PortType=blob  Muxed=off  Pose=off  Angle=on  AngleUnits=deg  ArcVelocity=off  ArcVelocityUnits=deg/s  ArcAcceleration=on  ArcAccelerationUnits=rad/s^2  CoordPosition=off  CoordPositionUnits=m  Velocity=off  VelocityUnits=m/s  Acceleration=on  AccelerationUnits=m/s^2  Quaternion=on  QuaternionDT=off  QuaternionDDT=off  QuaternionUnits=off  OutputVector=[ 3 3 ]  ActiveIO=off  Width=12  DialogClass=MechanicalSensorBlock  ReferenceFrame=Absolute (World)
  Bus Creator : BusCreator  Orientation=left  DialogController=Simulink.DDGSource_Bus  Inputs=6
  Corps : mblibv1/Bodies/Body  PhysicalDomain=mechanical  SubClassName=Unknown  LeftPortType=workingframe  RightPortType=workingframe  LConnTagsString=CS4|CS5|CS6|CS7|CG  RConnTagsString=CS1|CS2|CS3  DialogClass=MechanicalBodyBlock  Mass=Mecanique.Corps.Masse  MassUnits=kg  InertiaUnits=kg*m^2  Inertia=Mecanique.Corps.Inertie  Shape=Cylinder  ShapeDims=[1 1]  ShapeUnits=m  ShapeUse=false  Density=1  DensityUnits=kg/m^3  DensityUse=false  CG=Left$CG$[0 0 0]$ADJOINING$ADJOINING$m$[0 0 0]$Euler X-Y-Z$deg$ADJOINING$true  WorkingFrames=Right$CS1$[0 0 0]$CG$CG$m$[0 0 0]$Euler Z-Y-X$deg$CG$true#Right$CS2$[0 0 0]$CG$CG$m$[120 0 0]$Euler Z-Y-X$deg$CG$true#Right$CS3$[0 0 0]$CG$CG$m$[240 0 0]$Euler Z-Y-X$deg$CG$true#Left$CS4$[0 0 0]$CG$CG$m$[0 0 0]$Euler X-Y-Z$deg$WORLD$true#Left$CS5$[0 0 0]$CG$CG$m$[0 0 0]$Euler X-Y-Z$deg$WORLD$true#Left$CS6$[0 0 0]$CG$CG$m$[0 0 0]$Euler X-Y-Z$deg$WORLD$true#Left$CS7$[0 0 0]$CG$CG$m$[0 0 0]$Euler X-Y-Z$deg$WORLD$true
  Position : mblibv1/Sensors &  Actuators/Body Sensor  Orientation=left  Opaque=on  PhysicalDomain=Mechanical  PortType=blob  Muxed=off  Pose=on  Angle=on  AngleUnits=deg  ArcVelocity=off  ArcVelocityUnits=deg/s  ArcAcceleration=off  ArcAccelerationUnits=deg/s^2  CoordPosition=on  CoordPositionUnits=m  Velocity=off  VelocityUnits=m/s  Acceleration=off  AccelerationUnits=m/s^2  Quaternion=on  QuaternionDT=off  QuaternionDDT=off  QuaternionUnits=off  OutputVector=[ 3 9 ]  ActiveIO=off  Width=12  DialogClass=MechanicalSensorBlock  ReferenceFrame=Absolute (World)
  Vitesse : mblibv1/Sensors &  Actuators/Body Sensor  Orientation=left  Opaque=on  PhysicalDomain=Mechanical  PortType=blob  Muxed=off  Pose=off  Angle=on  AngleUnits=deg  ArcVelocity=on  ArcVelocityUnits=rad/s  ArcAcceleration=off  ArcAccelerationUnits=deg/s^2  CoordPosition=off  CoordPositionUnits=m  Velocity=on  VelocityUnits=m/s  Acceleration=off  AccelerationUnits=m/s^2  Quaternion=on  QuaternionDT=off  QuaternionDDT=off  QuaternionUnits=off  OutputVector=[ 3 3 ]  ActiveIO=off  Width=12  DialogClass=MechanicalSensorBlock  ReferenceFrame=Absolute (World)
  Bras1 : PMIOPort  Tag=PMCPort  Orientation=left  Port=1  Side=Left
  Air : PMIOPort  Tag=PMCPort  Port=2  Side=Right
  Bras2 : PMIOPort  Tag=PMCPort  Orientation=left  Port=3  Side=Left
  Environnement : PMIOPort  Tag=PMCPort  Port=4  Side=Right
  Bras3 : PMIOPort  Tag=PMCPort  Orientation=left  Port=5  Side=Left
  Position Vitesse Acceleration : Outport  Orientation=left
  wires:
  Position/1 -> Bus Creator/1  "xyz"
  Bus Creator/1 -> Position Vitesse Acceleration/1
  Position/2 -> Bus Creator/2  "dcm"
  Vitesse/1 -> Bus Creator/3  "x'y'z'"
  Vitesse/2 -> Bus Creator/4  "pqr"
  Body Sensor/1 -> Bus Creator/5  "x\"y\"z\""
  Body Sensor/2 -> Bus Creator/6  "p'q'r'"
  connections:
  Corps/RConn1 -- Bras1/RConn1
  Bras2/RConn1 -- Corps/RConn2
  Bras3/RConn1 -- Corps/RConn3
  Environnement/RConn1 -- Corps/LConn5
  Air/RConn1 -- Corps/LConn4
  Corps/LConn3 -- Body Sensor/LConn1
  Corps/LConn2 -- Vitesse/LConn1
  Position/LConn1 -- Corps/LConn1

== system drone/Mecanique1/Environnement ==
  note: POUR VISUALISER
  Ground : mblibv1/Bodies/Ground  Opaque=on  LeftPortType=env  RightPortType=workingframe  PhysicalDomain=Mechanical  DialogClass=GroundBlock  CoordPosition=[0 0 0]  CoordPositionUnits=m  StateVectorMgrId=-1  MachineId=[0 0]  ShowEnvPort=on
  Machine Environment : mblibv1/Bodies/Machine Environment  Tag=Factory ground  DialogController=MECH.DialogSource  Opaque=on  PortType=env  PhysicalDomain=Mechanical  DialogTemplateClass=MECH.MachineEnvironment  SyncWhenCopied=off  Gravity=Environnement.Gravite  GravityUnits=m/s^2  GravityAsSignal=off  Dimensionality=3D Only  AnalysisType=Forward dynamics  LinearAssemblyTolerance=1e-3  LinearAssemblyToleranceUnits=m  AngularAssemblyTolerance=1e-3  AngularAssemblyToleranceUnits=rad  ConstraintSolverType=Stabilizing  ConstraintRelTolerance=1e-4  ConstraintAbsTolerance=1e-4  UseRobustSingularityHandling=off  StatePerturbationType=Fixed  PerturbationSize=1e-5  VisualizeMachine=on
  Six-DoF : mblibv1/Joints/Six-DoF  PhysicalDomain=mechanical  SubClassName=Unknown  LeftPortType=blob  RightPortType=blob  LConnTagsString=__newl0  RConnTagsString=__newr0  NumSAPorts=0  CutJoint=off  MarkAsCut=off  Primitives=prismatic_prismatic_prismatic_spherical  PrimitiveProps=P1$INERTIAL$[1 0 0]$prismatic#P2$INERTIAL$[0 1 0]$prismatic#P3$INERTIAL$[0 0 1]$prismatic#S$INERTIAL$[0 0 0]$spherical  DialogClass=JointBlock
  Corps : PMIOPort  Tag=PMCPort  Orientation=left  Port=1  Side=Left
  connections:
  Ground/RConn1 -- Six-DoF/LConn1
  Six-DoF/RConn1 -- Corps/RConn1
  Machine Environment/RConn1 -- Ground/LConn1

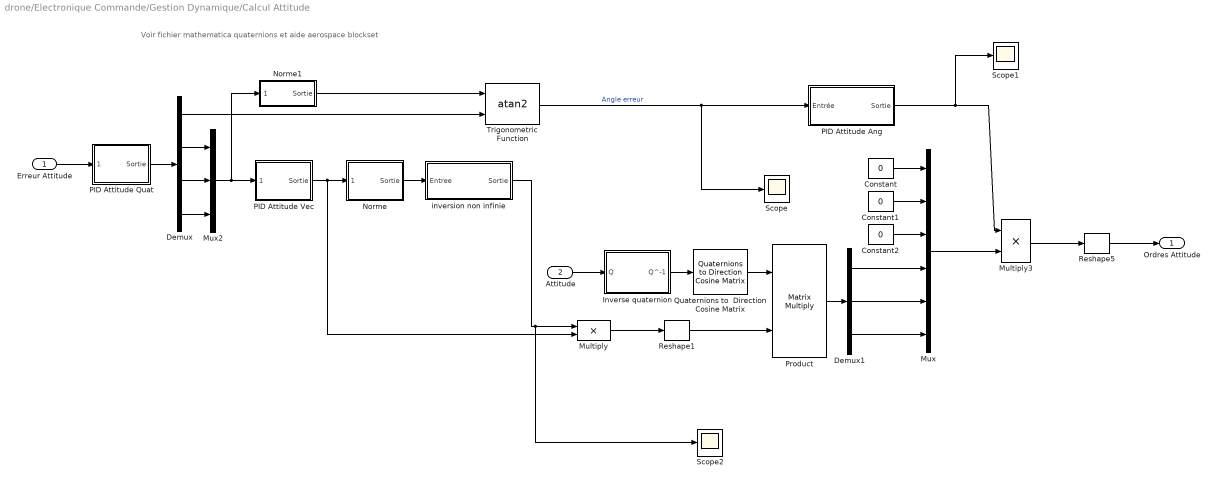
== system drone/Electronique Commande/Gestion Dynamique/Calcul Attitude ==
  note: Voir fichier mathematica quaternions et aide aerospace blockset
  Erreur Attitude : Inport  Port=1  LatchInput=off
  Attitude : Inport  Port=2  LatchInput=off
  Constant : Constant  Value=0
  Constant1 : Constant  Value=0
  Constant2 : Constant  Value=0
  Demux : Demux
  Demux1 : Demux  Outputs=3
  Inverse quaternion : Subsystem
  Multiply : Product  Inputs=**  OutScaling=2^-10
  Multiply3 : Product  Inputs=**  OutScaling=2^-10
  Mux : Mux  Inputs=6
  Mux2 : Mux  Inputs=3
  Norme : Subsystem
  Norme1 : Subsystem
  PID Attitude Ang : Subsystem
  PID Attitude Quat : Subsystem
  PID Attitude Vec : Subsystem
  Product : Product  Multiplication=Matrix(*)  RndMeth=Zero
  Quaternions to  Direction Cosine Matrix : aerolibtransform2/Quaternions to  Direction Cosine Matrix
  Reshape1 : simulink/Math Operations/Reshape  OutputDimensionality=1-D array  OutputDimensions=[1,1]
  Reshape5 : simulink/Math Operations/Reshape  OutputDimensionality=1-D array  OutputDimensions=[1,1]
  Scope : Scope
      settings: SaveName=ScopeData5
  Scope1 : Scope
      settings: YMax=37.5  SaveName=ScopeData7
  Scope2 : Scope
      settings: YMin=0  YMax=1.4e+013  SaveName=ScopeData9
  Trigonometric Function : Trigonometry  Operator=atan2
  inversion non infinie : Subsystem
  Ordres Attitude : Outport
      settings: BusObject=perturbations
  wires:
  Constant/1 -> Mux/1
  Constant1/1 -> Mux/2
  Constant2/1 -> Mux/3
  Norme/1(Sortie) -> inversion non infinie/1(Entree)
  Mux/1 -> Multiply3/2
  Multiply3/1 -> Reshape5/1
  Reshape5/1 -> Ordres Attitude/1
  Quaternions to  Direction Cosine Matrix/1 -> Product/1
  Reshape1/1 -> Product/2
  Product/1 -> Demux1/1
  Demux1/1 -> Mux/4
  Demux1/2 -> Mux/5
  Demux1/3 -> Mux/6
  Demux/1 -> Trigonometric Function/2
  Trigonometric Function/1 -> Scope/1, PID Attitude Ang/1(Entrée)  "Angle erreur"
  Multiply/1 -> Reshape1/1
  inversion non infinie/1(Sortie) -> Multiply/1, Scope2/1
  Inverse quaternion/1(Q^-1) -> Quaternions to  Direction Cosine Matrix/1
  Attitude/1 -> Inverse quaternion/1(Q)
  Erreur Attitude/1 -> PID Attitude Quat/1(Entrée)
  PID Attitude Ang/1(Sortie) -> Multiply3/1, Scope1/1
  Demux/2 -> Mux2/1
  Demux/3 -> Mux2/2
  Demux/4 -> Mux2/3
  Mux2/1 -> PID Attitude Vec/1(Entrée), Norme1/1(Entrée)
  PID Attitude Vec/1(Sortie) -> Norme/1(Entrée), Multiply/2
  Norme1/1(Sortie) -> Trigonometric Function/1
  PID Attitude Quat/1(Sortie) -> Demux/1
